simulink model "uavCtrlcp"  (R2018b)
settings: Solver=VariableStepAuto  StartTime=0.0  StopTime=10  RelTol=1e-3  EnableMultiTasking=on
values from neighbouring files (symbols this model uses):
  alate = [-0.828295210678 -580.980828285 93.7619059623 0 0 34.9999999994 0.00784601123454 -40.6126483821 -0.583194393032 1 0 0 ... (36 elements, 6x6)]    [data.mat]
  along = [-0.0755841369079 -0.0159993821818 -1.16199905251e-15 0 7.70988211545e-14 3.71213864216 -6.99491543237 -75.8557513579 0 -34.9999999994 -4.92343950828e-13 1 ... (25 elements, 5x5)]    [data.mat]
  blate = [0  0; -6.11443709175  -0.243360680269; 0.0919199677882  -0.772963365492; 0  0; 0  0; 0  0]    [data.mat]
  blong = [2.20949307472e-13  0.0245242451103; -0.00965326437836  -5.49781215794e-06; -1.41495298524  0; 0  0; 0  0]    [data.mat]
  clate = [57.2957795131 0 0 0 0 0 0 57.2957795131 0 0 0 0 ... (36 elements, 6x6)]    [data.mat]
  clong = [1 0 0 0 0 0 57.2957795131 0 0 0 0 0 ... (25 elements, 5x5)]    [data.mat]
  dlate = [0  0; 0  0; 0  0; 0  0; 0  0; 0  0]    [data.mat]
  dlong = [0  0; 0  0; 0  0; 0  0; 0  0]    [data.mat]
  utrim = [1.49457502486 3.95000888139e-15 -4.35170409107e-15 53.9352950493]    [data.mat]
settings Model: Creator=Administrator  LastModifiedBy=win-s
settings DataIOCC: LimitDataPoints=on  SaveFormat=Array  SignalLoggingSaveFormat=ModelDataLogs
settings OptimizationCC: ExpressionDepthLimit=2147483647  InitFltsAndDblsToZero=on  LifeSpan=inf
settings DebuggingCC: UnderspecifiedInitializationDetection=Classic  MergeDetectMultiDrivingBlocksExec=none  SolverPrmCheckMsg=warning  FcnCallInpInsideContextMsg=warning  StateNameClashWarn=warning  SFUnexpectedBacktrackingDiag=warning  SFNoUnconditionalDefaultTransitionDiag=warning
settings HardwareCC: ProdBitPerPointer=32  ProdBitPerSizeT=32  ProdBitPerPtrDiffT=32  ProdLargestAtomicFloat=None  ProdIntDivRoundTo=Undefined  ProdEndianess=Unspecified  ProdWordSize=32  ProdHWDeviceType=32-bit Generic
settings ModelReferenceCC: PropagateSignalLabelsOutOfModel=off
settings SFSimCC: SimUseLocalCustomCode=off
settings RTWCC: RTWUseLocalCustomCode=off
settings CodeAppCC: StateflowObjectComments=on
settings GRTTargetCC: TargetLangStandard=C89/C90 (ANSI)  CombineOutputUpdateFcns=off  GRTInterface=on
settings ConfigComp: CovMetricSettings=dw  CovHtmlReporting=on  CovSaveCumulativeToWorkspaceVar=on  CovSaveSingleToWorkspaceVar=on  CovExternalEMLEnable=off

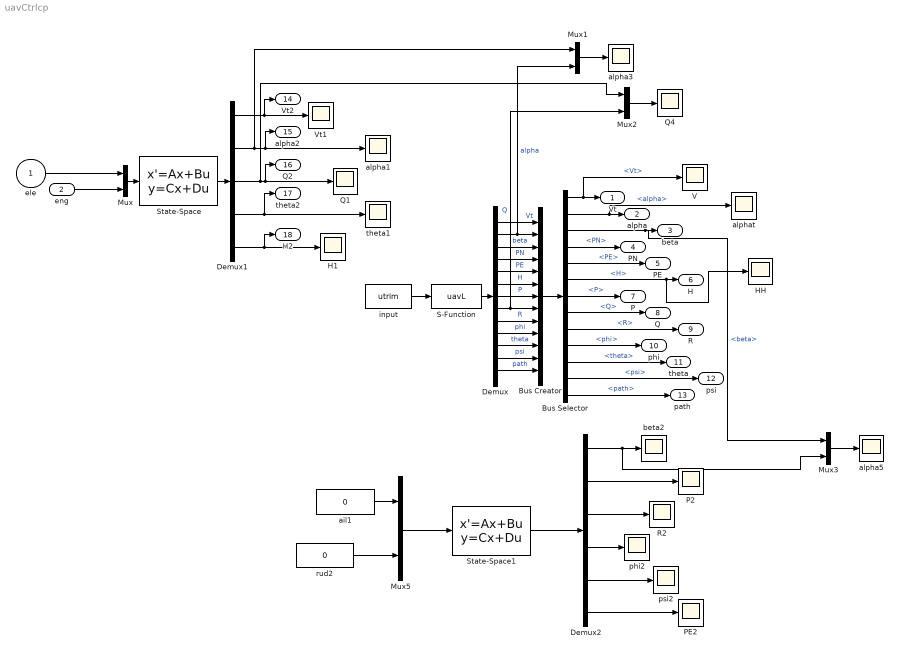
== system uavCtrlcp ==
  ele : Inport
  eng : Inport  Port=2
  Bus Creator : BusCreator  Inputs=13
  Bus Selector : BusSelector  OutputSignals=Vt,alpha,beta,PN,PE,H,P,Q,R,phi,theta,psi,path
  Demux : Demux  Outputs=13
  Demux1 : Demux  Outputs=5
  Demux2 : Demux  Outputs=6
  H1 : Scope
  HH : Scope
  Mux{,1..3,5} (5 alike) : Mux  Inputs=2
  P2 : Scope
  PE2 : Scope
  Q1 : Scope
  Q4 : Scope
  R2 : Scope
  S-Function : S-Function  FunctionName=uavL  SFunctionDeploymentMode=off  EnableBusSupport=off
  State-Space : StateSpace  A=along  B=blong  C=clong  D=dlong  InitialCondition=[0 1*pi/180 0 0 0]
  State-Space1 : StateSpace  A=alate  B=blate  C=clate  D=dlate  InitialCondition=[1*pi/180 0 0 0 0 0]
  V : Scope
  Vt1 : Scope
  ail1 : Constant  Value=0
  alpha1 : Scope
  alpha3 : Scope
  alpha5 : Scope
  alphat : Scope
  beta2 : Scope
  input : Constant  Value=utrim
  phi2 : Scope
  psi2 : Scope
  rud2 : Constant  Value=0
  theta1 : Scope
  Vt : Outport
  alpha : Outport  Port=2
  beta : Outport  Port=3
  PN : Outport  Port=4
  PE : Outport  Port=5
  H : Outport  Port=6
  P : Outport  Port=7
  Q : Outport  Port=8
  R : Outport  Port=9
  phi : Outport  Port=10
  theta : Outport  Port=11
  psi : Outport  Port=12
  path : Outport  Port=13
  Vt2 : Outport  Port=14
  alpha2 : Outport  Port=15
  Q2 : Outport  Port=16
  theta2 : Outport  Port=17
  H2 : Outport  Port=18
  wires:
  S-Function/1 -> Demux/1
  Demux/1 -> Bus Creator/1  "Vt"
  Demux/2 -> Mux1/2, Bus Creator/2  "alpha"
  Demux/3 -> Bus Creator/3  "beta"
  Demux/4 -> Bus Creator/4  "PN"
  Demux/5 -> Bus Creator/5  "PE"
  Demux/6 -> Bus Creator/6  "H"
  Demux/7 -> Bus Creator/7  "P"
  Demux/8 -> Mux2/2, Bus Creator/8  "Q"
  Demux/9 -> Bus Creator/9  "R"
  Demux/10 -> Bus Creator/10  "phi"
  Demux/11 -> Bus Creator/11  "theta"
  Demux/12 -> Bus Creator/12  "psi"
  Demux/13 -> Bus Creator/13  "path"
  Bus Creator/1 -> Bus Selector/1
  Bus Selector/1 -> V/1, Vt/1  "<Vt>"
  Bus Selector/2 -> alphat/1, alpha/1  "<alpha>"
  Bus Selector/3 -> Mux3/1, beta/1  "<beta>"
  Bus Selector/4 -> PN/1  "<PN>"
  Bus Selector/13 -> path/1  "<path>"
  Bus Selector/12 -> psi/1  "<psi>"
  Bus Selector/11 -> theta/1  "<theta>"
  Bus Selector/10 -> phi/1  "<phi>"
  Bus Selector/9 -> R/1  "<R>"
  Bus Selector/8 -> Q/1  "<Q>"
  Bus Selector/7 -> P/1  "<P>"
  Bus Selector/6 -> HH/1, H/1  "<H>"
  Bus Selector/5 -> PE/1  "<PE>"
  input/1 -> S-Function/1
  Mux/1 -> State-Space/1
  Demux1/1 -> Vt2/1, Vt1/1
  Demux1/2 -> Mux1/1, alpha2/1, alpha1/1
  Demux1/3 -> Mux2/1, Q2/1, Q1/1
  Demux1/4 -> theta2/1, theta1/1
  Demux1/5 -> H2/1, H1/1
  State-Space/1 -> Demux1/1
  eng/1 -> Mux/2
  ele/1 -> Mux/1
  Mux1/1 -> alpha3/1
  Mux2/1 -> Q4/1
  Demux2/1 -> Mux3/2, beta2/1
  Demux2/2 -> P2/1
  Demux2/3 -> R2/1
  Demux2/4 -> phi2/1
  Demux2/5 -> psi2/1
  State-Space1/1 -> Demux2/1
  Demux2/6 -> PE2/1
  ail1/1 -> Mux5/1
  Mux5/1 -> State-Space1/1
  rud2/1 -> Mux5/2
  Mux3/1 -> alpha5/1
